simulink model "durumi2_sim"  (R2022a)
settings: Solver=ode4  StartTime=0.0  StopTime=50  FixedStep=0.01  RelTol=1e-5  EnableMultiTasking=on
values from neighbouring files (symbols this model uses):
  u0 = op.Inputs.u    [cal_trim_durumi2.m]
  u_da = 0    [cal_trim_durumi2.m]
  u_de = 0    [cal_trim_durumi2.m]
  u_dr = 0    [cal_trim_durumi2.m]
  u_th = 0    [cal_trim_durumi2.m]
undefined symbols (not defined in the file or in its folder): sigbuilder_block
libraries: simulink_extras x3
settings Model: Creator=김응태  LastModifiedBy=김응태
settings DataIOCC: SaveFormat=Array  SignalLoggingSaveFormat=ModelDataLogs  ReturnWorkspaceOutputs=off  SignalLoggingName=sigsOut
settings OptimizationCC: BooleanDataType=off
settings DebuggingCC: SaveWithParameterizedLinksMsg=none  UnderspecifiedInitializationDetection=Classic  MergeDetectMultiDrivingBlocksExec=none  SignalResolutionControl=TryResolveAllWithWarning  MultiTaskDSMMsg=warning  MultiTaskCondExecSysMsg=none  UnconnectedInputMsg=warning  UnconnectedOutputMsg=warning  UnconnectedLineMsg=warning
settings HardwareCC: ProdBitPerPointer=32  ProdBitPerSizeT=32  ProdBitPerPtrDiffT=32  ProdLargestAtomicFloat=None  ProdIntDivRoundTo=Undefined  ProdEndianess=Unspecified  ProdWordSize=32  ProdHWDeviceType=32-bit Generic  TargetUnknown=on
settings ModelReferenceCC: PropagateSignalLabelsOutOfModel=off
settings GRTTargetCC: CombineOutputUpdateFcns=off  GRTInterface=on
settings ConfigComp: CovMetricSettings=dw  CovSaveCumulativeToWorkspaceVar=on  CovSaveSingleToWorkspaceVar=on

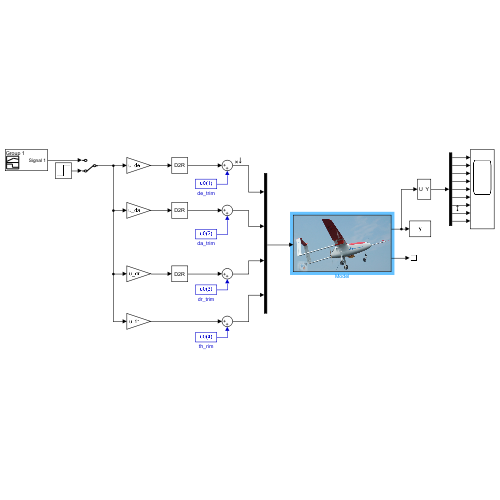
[thumbnail: Simulink's stored preview of the top-level diagram]
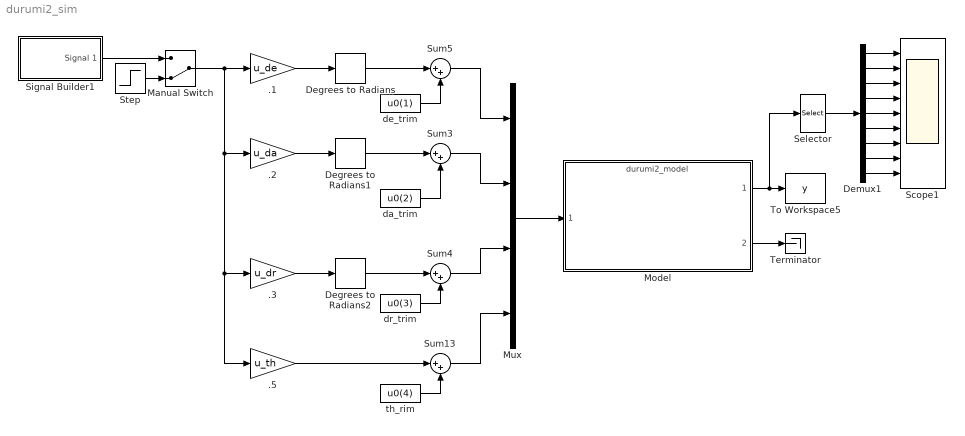
== system durumi2_sim ==
  .1 : Gain  Gain=u_de  OutDataTypeStr=Inherit: Same as input  ParamDataTypeStr=Inherit: Same as input
  .2 : Gain  Gain=u_da  OutDataTypeStr=Inherit: Same as input  ParamDataTypeStr=Inherit: Same as input
  .3 : Gain  Gain=u_dr  OutDataTypeStr=Inherit: Same as input  ParamDataTypeStr=Inherit: Same as input
  .5 : Gain  Gain=u_th  OutDataTypeStr=Inherit: Same as input  ParamDataTypeStr=Inherit: Same as input
  Degrees to Radians : simulink_extras/Transformations/Degrees to Radians
  Degrees to Radians1 : simulink_extras/Transformations/Degrees to Radians
  Degrees to Radians2 : simulink_extras/Transformations/Degrees to Radians
  Demux1 : Demux  Outputs=9
  Manual Switch : ManualSwitch  CurrentSetting=0
  Model : ModelReference  ModelNameDialog=durumi2_model.slx  SimulationMode=Normal  ModelReferenceVersion=1.71
      mask Display: image('durumi2.PNG'); % Use "Edit Image" on toolstrip to change.
  Mux : Mux
  Scope1 : Scope  NumInputPorts=9
  Selector : Selector  InputPortWidth=12  IndexOptions=Index vector (dialog)  Indices=[1:9]  OutputSizes=1
  Signal Builder1 : Subsystem  Tag=STV Subsys  LoadFcn=sigbuilder_block('load');  StartFcn=sigbuilder_block('start');  StopFcn=sigbuilder_block('stop');  ClipboardFcn=sigbuilder_block('clipboard');  mask(Sigbuilder block){tuvar=[0:10]}
      mask help: Simulink:masks:SigbuilderBlock_MD
      mask init:
      | if ~strcmp(get_param(bdroot(gcbh),'SimulationStatus'),'stopped') tuvar = sigbuilder_block('maskInit'); end
      settings: CopyFcn=sigbuilder_block('copy');  DeleteFcn=sigbuilder_block('delete');  ModelCloseFcn=sigbuilder_block('modelClose');  PreSaveFcn=sigbuilder_block('preSave');  PauseFcn=sigbuilder_block('pause');  ContinueFcn=sigbuilder_block('continue');  NameChangeFcn=sigbuilder_block('namechange');  OpenFcn=sigbuilder_block('open',[437.6 199.2 550.4 400 ]);  CloseFcn=sigbuilder_block('close');
      mask Display: plot(0, 0, 100, 100,[2, 2, 32, 32, 2], [68, 8, 8, 68, 68],[32, 2], [38, 38], [32, 19, 2],[53, 60, 44], [32, 17, 17, 2],[16, 16, 31, 31]);txt = getActiveGroup(gcbh);text(2, 100, txt,'verticalAlignment', 'top');
  Step : Step  SampleTime=0
  Sum{3..5,13} (4 alike) : Sum  Inputs=|++  InputSameDT=on  OutDataTypeStr=Inherit: Same as first input
  Terminator : Terminator
  To Workspace5 : ToWorkspace  VariableName=y  SampleTime=-1
  da_trim : Constant  Value=u0(2)  VectorParams1D=off
  de_trim : Constant  Value=u0(1)  VectorParams1D=off
  dr_trim : Constant  Value=u0(3)  VectorParams1D=off
  th_rim : Constant  Value=u0(4)  VectorParams1D=off
  wires:
  Model/1 -> To Workspace5/1, Selector/1
  .3/1 -> Degrees to Radians2/1
  Step/1 -> Manual Switch/2
  .1/1 -> Degrees to Radians/1
  .5/1 -> Sum13/1
  Sum3/1 -> Mux/2
  Sum13/1 -> Mux/4
  da_trim/1 -> Sum3/2
  th_rim/1 -> Sum13/2
  dr_trim/1 -> Sum4/2
  .2/1 -> Degrees to Radians1/1
  de_trim/1 -> Sum5/2
  Sum4/1 -> Mux/3
  Sum5/1 -> Mux/1
  Mux/1 -> Model/1
  Selector/1 -> Demux1/1
  Demux1/8 -> Scope1/8
  Demux1/7 -> Scope1/7
  Demux1/6 -> Scope1/6
  Demux1/4 -> Scope1/4
  Demux1/3 -> Scope1/3
  Demux1/2 -> Scope1/2
  Demux1/1 -> Scope1/1
  Demux1/5 -> Scope1/5
  Demux1/9 -> Scope1/9
  Manual Switch/1 -> .2/1, .3/1, .5/1, .1/1
  Signal Builder1/1(Signal 1) -> Manual Switch/1
  Model/2 -> Terminator/1
  Degrees to Radians/1 -> Sum5/1
  Degrees to Radians1/1 -> Sum3/1
  Degrees to Radians2/1 -> Sum4/1

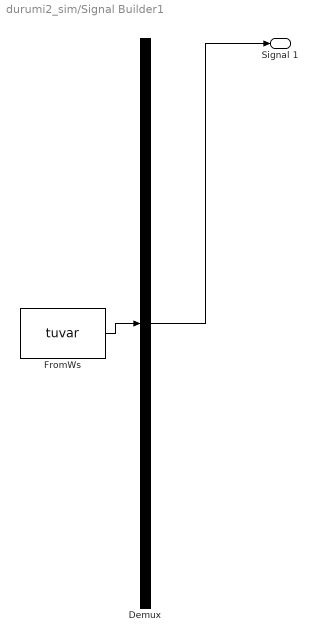
== system durumi2_sim/Signal Builder1 ==
  Demux : Demux  Tag=STV Demux  Outputs=1
      settings: DisplayOption=none
  FromWs : FromWorkspace  Tag=STV FromWs  VariableName=tuvar
      SigBuilderData=|
      | common.afterFinalStr = 'Extrapolate'
      | common.sampleTime = 0
      | dataSet.timeRange = [0 10]
      | dataSet.name = 'Group 1'
      | sbobj.Groups.Name = 'Group 1'
      | sbobj.Groups.Signals.Name = 'Signal 1'
      | sbobj.Groups.Signals.XData = [0 4 4 6 6 10]
      | sbobj.Groups.Signals.YData = [0 0 1 1 0 0]
  Signal 1 : Outport  Tag=STV Outport
  wires:
  FromWs/1 -> Demux/1
  Demux/1 -> Signal 1/1
